simulink model "qvm_bocsh"  (Simulink 4.0)
settings: Solver=ode45  StartTime=0.0  StopTime=5.0  MaxStep=0.001  RelTol=1e-4
undefined symbols (not defined in the file): Z10
libraries: simulink_extras x7, dtlib x1
(part 2 of 2)

== system qvm_bocsh/ABS Block/Signal Processing/Subsystem3 ==
  In1 : Inport  Port=1  PortDimensions=-1  SampleTime=-1  DataType=auto
      settings: SignalType=auto
  Logical Operator2 : Logic  Operator=XOR  Inputs=2
  Logical Operator3 : Logic  Operator=AND  Inputs=2
  Memory : Memory  X0=0  InheritSampleTime=off
  Pos. Slope : Outport  Port=1
  wires:
  Logical Operator3/1 -> Pos. Slope/1
  In1/1 -> Logical Operator2/2, Memory/1, Logical Operator3/1
  Logical Operator2/1 -> Logical Operator3/2
  Memory/1 -> Logical Operator2/1

== system qvm_bocsh/ABS Block/Signal Processing/Subsystem5 ==
  In1 : Inport  Port=1  PortDimensions=-1  SampleTime=-1  DataType=auto
      settings: SignalType=auto
  Logical Operator2 : Logic  Operator=XOR  Inputs=2
  Logical Operator3 : Logic  Operator=AND  Inputs=2
  Memory : Memory  X0=0  InheritSampleTime=off
  Pos. Slope : Outport  Port=1
  wires:
  Logical Operator3/1 -> Pos. Slope/1
  In1/1 -> Logical Operator2/2, Memory/1, Logical Operator3/1
  Logical Operator2/1 -> Logical Operator3/2
  Memory/1 -> Logical Operator2/1

== system qvm_bocsh/ABS Block/Signal Processing/Subsystem7 ==
  In1 : Inport  Port=1  PortDimensions=-1  SampleTime=-1  DataType=auto
      settings: SignalType=auto
  Logical Operator2 : Logic  Operator=XOR  Inputs=2
  Logical Operator3 : Logic  Operator=AND  Inputs=2
  Memory : Memory  X0=0  InheritSampleTime=off
  Neg. Slope : Outport  Port=1
  wires:
  Logical Operator3/1 -> Neg. Slope/1
  In1/1 -> Logical Operator2/2, Memory/1
  Logical Operator2/1 -> Logical Operator3/2
  Memory/1 -> Logical Operator3/1, Logical Operator2/1

== system qvm_bocsh/ABS Block/Signal Processing/Subsystem8 ==
  In1 : Inport  Port=1  PortDimensions=-1  SampleTime=-1  DataType=auto
      settings: SignalType=auto
  Logical Operator2 : Logic  Operator=XOR  Inputs=2
  Logical Operator3 : Logic  Operator=AND  Inputs=2
  Memory : Memory  X0=0  InheritSampleTime=off
  Neg. Slope : Outport  Port=1
  wires:
  Logical Operator3/1 -> Neg. Slope/1
  In1/1 -> Logical Operator2/2, Memory/1
  Logical Operator2/1 -> Logical Operator3/2
  Memory/1 -> Logical Operator3/1, Logical Operator2/1

== system qvm_bocsh/ABS Block/Signal Processing/Subsystem9 ==
  In1 : Inport  Port=1  PortDimensions=-1  SampleTime=-1  DataType=auto
      settings: SignalType=auto
  Logical Operator2 : Logic  Operator=XOR  Inputs=2
  Logical Operator3 : Logic  Operator=AND  Inputs=2
  Memory : Memory  X0=0  InheritSampleTime=off
  Pos. Slope : Outport  Port=1
  wires:
  Logical Operator3/1 -> Pos. Slope/1
  In1/1 -> Logical Operator2/2, Memory/1, Logical Operator3/1
  Logical Operator2/1 -> Logical Operator3/2
  Memory/1 -> Logical Operator2/1

== system qvm_bocsh/ABS Block/Signal Processing/Threshold  A, +a ==
  Om_dot_periph. : Inport  Port=1  PortDimensions=-1  SampleTime=-1  DataType=auto
      settings: SignalType=auto
  +a Comparator1 : RelationalOperator  Operator=>
  +a positive acc. : Constant  Orientation=left  Value=pos_a
  A Comparator : RelationalOperator  Operator=>
  A positive acc. : Constant  Orientation=left  Value=A
  " > A" : Outport  Port=1
  > +a : Outport  Port=2
  wires:
  +a Comparator1/1 -> > +a/1
  +a positive acc./1 -> +a Comparator1/2
  A Comparator/1 -> " > A"/1
  A positive acc./1 -> A Comparator/2
  Om_dot_periph./1 -> A Comparator/1, +a Comparator1/1

== system qvm_bocsh/ABS Block/Signal Processing/Threshold -a ==
  Om_dot_periph. : Inport  Port=1  PortDimensions=-1  SampleTime=-1  DataType=auto
      settings: SignalType=auto
  -a Comparator1 : RelationalOperator  Operator=>=
  -a negative acc. : Constant  Orientation=left  Value=neg_a
  Gain2 : Gain  Gain=-1  Multiplication=Element-wise(K.*u)  SaturateOnIntegerOverflow=on
  > -a : Outport  Port=1
  wires:
  Gain2/1 -> -a Comparator1/1
  -a Comparator1/1 -> > -a/1
  -a negative acc./1 -> -a Comparator1/2
  Om_dot_periph./1 -> Gain2/1

== system qvm_bocsh/ABS Block/Subsystem/Generator ==
  In : Inport  Port=1  PortDimensions=-1  SampleTime=-1  DataType=auto
      settings: SignalType=auto
  Constant1 : Constant  Orientation=left  Value=0
  Data Type Conversion1 : DataTypeConversion  DataType=boolean  SaturateOnIntegerOverflow=on
  Data Type Conversion2 : DataTypeConversion  Orientation=left  DataType=double  SaturateOnIntegerOverflow=on
  Data Type Conversion5 : DataTypeConversion  DataType=boolean  SaturateOnIntegerOverflow=on
  Logical Operator2 : Logic  Operator=OR  Inputs=2
  Memory1 : Memory  Orientation=left  X0=0  InheritSampleTime=off
  Memory2 : Memory  Orientation=left  X0=0  InheritSampleTime=off
  Subsystem2 : Subsystem  SimViewingDevice=off
      settings: Permissions=ReadWrite  RTWFcnNameOpts=Auto  RTWFileNameOpts=Auto
  Switch2 : Switch  Threshold=1
  Timer R1 : Subsystem  SimViewingDevice=off  mask{TC=TC}
      mask prompts: TC "Cycle Time [s]"
      settings: Permissions=ReadWrite  RTWFcnNameOpts=Auto  RTWFileNameOpts=Auto
  Timer R2 : Subsystem  SimViewingDevice=off  mask{TO=TO}
      mask prompts: TO "Open time [s]"
      settings: Permissions=ReadWrite  RTWFcnNameOpts=Auto  RTWFileNameOpts=Auto
  Out : Outport  Port=1
  wires:
  Timer R2/1(Time elapse) -> Out/1
  Data Type Conversion2/1 -> Switch2/1
  Data Type Conversion1/1 -> Logical Operator2/2
  Constant1/1 -> Switch2/3
  Memory2/1 -> Data Type Conversion2/1
  Switch2/1 -> Data Type Conversion1/1
  Memory1/1 -> Memory2/1, Timer R2/2(Reset), Timer R1/2(Reset)
  Data Type Conversion5/1 -> Switch2/2, Subsystem2/1(In1)
  Subsystem2/1(Pos. Slpoe) -> Logical Operator2/1
  In/1 -> Data Type Conversion5/1
  Timer R1/1(Time elapse) -> Memory1/1
  Logical Operator2/1 -> Timer R1/1(Start), Timer R2/1(Start)

== system qvm_bocsh/ABS Block/Subsystem/One Cycle Indicator ==
  In : Inport  Port=1  PortDimensions=-1  SampleTime=-1  DataType=auto
      settings: SignalType=auto
  Logical Operator3 : Logic  Operator=OR  Inputs=2
  Memory : Memory  X0=0  InheritSampleTime=off
  S-R Flip-Flop : simulink_extras/Flip Flops/S-R Flip-Flop  Orientation=left  initial_condition=0
  Terminator : Terminator
  Q : Outport  Port=1
  wires:
  S-R Flip-Flop/2 -> Terminator/1
  In/1 -> Logical Operator3/2
  S-R Flip-Flop/1 -> Memory/1
  Memory/1 -> Q/1, Logical Operator3/1
  Logical Operator3/1 -> S-R Flip-Flop/1

== system qvm_bocsh/ABS Block/Subsystem/Generator/Subsystem2 ==
  In1 : Inport  Port=1  PortDimensions=-1  SampleTime=-1  DataType=auto
      settings: SignalType=auto
  Logical Operator2 : Logic  Operator=XOR  Inputs=2
  Logical Operator3 : Logic  Operator=AND  Inputs=2
  Memory : Memory  X0=0  InheritSampleTime=off
  Pos. Slpoe : Outport  Port=1
  wires:
  Logical Operator3/1 -> Pos. Slpoe/1
  In1/1 -> Logical Operator3/1, Memory/1, Logical Operator2/2
  Logical Operator2/1 -> Logical Operator3/2
  Memory/1 -> Logical Operator2/1

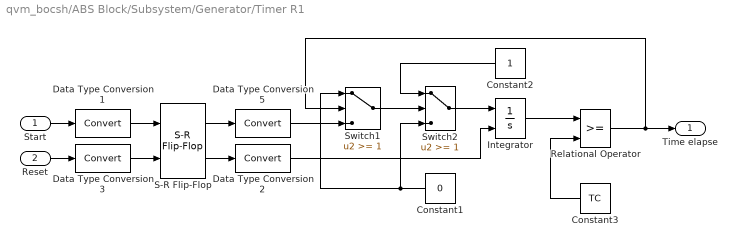
== system qvm_bocsh/ABS Block/Subsystem/Generator/Timer R1 ==
  Start : Inport  Port=1  PortDimensions=-1  SampleTime=-1  DataType=auto
      settings: SignalType=auto
  Reset : Inport  Port=2  PortDimensions=-1  SampleTime=-1  DataType=auto
      settings: SignalType=auto
  Constant1 : Constant  Orientation=left  Value=0
  Constant2 : Constant  Orientation=left  Value=1
  Constant3 : Constant  Orientation=left  Value=TC
  Data Type Conversion1 : DataTypeConversion  DataType=boolean  SaturateOnIntegerOverflow=on
  Data Type Conversion2 : DataTypeConversion  DataType=double  SaturateOnIntegerOverflow=on
  Data Type Conversion3 : DataTypeConversion  DataType=boolean  SaturateOnIntegerOverflow=on
  Data Type Conversion5 : DataTypeConversion  DataType=double  SaturateOnIntegerOverflow=on
  Integrator : Integrator  ExternalReset=level  InitialConditionSource=internal  InitialCondition=0  LimitOutput=off  UpperSaturationLimit=inf  LowerSaturationLimit=-inf  ShowSaturationPort=off  ShowStatePort=off  AbsoluteTolerance=auto
  Relational Operator : RelationalOperator  Operator=>=
  S-R Flip-Flop : simulink_extras/Flip Flops/S-R Flip-Flop  initial_condition=0
  Switch1 : Switch  Threshold=1
  Switch2 : Switch  Threshold=1
  Time elapse : Outport  Port=1
  wires:
  Data Type Conversion5/1 -> Switch1/3
  S-R Flip-Flop/1 -> Data Type Conversion5/1
  Data Type Conversion2/1 -> Integrator/2
  S-R Flip-Flop/2 -> Data Type Conversion2/1
  Start/1 -> Data Type Conversion1/1
  Data Type Conversion1/1 -> S-R Flip-Flop/1
  Reset/1 -> Data Type Conversion3/1
  Data Type Conversion3/1 -> S-R Flip-Flop/2
  Switch2/1 -> Integrator/1
  Constant3/1 -> Relational Operator/2
  Constant1/1 -> Switch1/1, Switch2/3
  Integrator/1 -> Relational Operator/1
  Relational Operator/1 -> Switch1/2, Time elapse/1
  Switch1/1 -> Switch2/2
  Constant2/1 -> Switch2/1

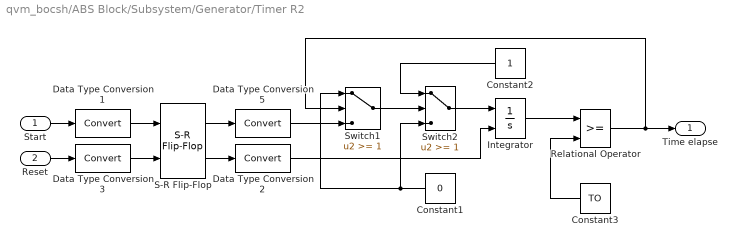
== system qvm_bocsh/ABS Block/Subsystem/Generator/Timer R2 ==
  Start : Inport  Port=1  PortDimensions=-1  SampleTime=-1  DataType=auto
      settings: SignalType=auto
  Reset : Inport  Port=2  PortDimensions=-1  SampleTime=-1  DataType=auto
      settings: SignalType=auto
  Constant1 : Constant  Orientation=left  Value=0
  Constant2 : Constant  Orientation=left  Value=1
  Constant3 : Constant  Orientation=left  Value=TO
  Data Type Conversion1 : DataTypeConversion  DataType=boolean  SaturateOnIntegerOverflow=on
  Data Type Conversion2 : DataTypeConversion  DataType=double  SaturateOnIntegerOverflow=on
  Data Type Conversion3 : DataTypeConversion  DataType=boolean  SaturateOnIntegerOverflow=on
  Data Type Conversion5 : DataTypeConversion  DataType=double  SaturateOnIntegerOverflow=on
  Integrator : Integrator  ExternalReset=level  InitialConditionSource=internal  InitialCondition=0  LimitOutput=off  UpperSaturationLimit=inf  LowerSaturationLimit=-inf  ShowSaturationPort=off  ShowStatePort=off  AbsoluteTolerance=auto
  Relational Operator : RelationalOperator  Operator=>=
  S-R Flip-Flop : simulink_extras/Flip Flops/S-R Flip-Flop  initial_condition=0
  Switch1 : Switch  Threshold=1
  Switch2 : Switch  Threshold=1
  Time elapse : Outport  Port=1
  wires:
  Data Type Conversion5/1 -> Switch1/3
  S-R Flip-Flop/1 -> Data Type Conversion5/1
  Data Type Conversion2/1 -> Integrator/2
  S-R Flip-Flop/2 -> Data Type Conversion2/1
  Start/1 -> Data Type Conversion1/1
  Data Type Conversion1/1 -> S-R Flip-Flop/1
  Reset/1 -> Data Type Conversion3/1
  Data Type Conversion3/1 -> S-R Flip-Flop/2
  Switch2/1 -> Integrator/1
  Constant3/1 -> Relational Operator/2
  Constant1/1 -> Switch1/1, Switch2/3
  Integrator/1 -> Relational Operator/1
  Relational Operator/1 -> Switch1/2, Time elapse/1
  Switch1/1 -> Switch2/2
  Constant2/1 -> Switch2/1
